simulink subsystem "Spline_Path_Following_sub"  (R2023b)
settings: Solver=VariableStepAuto  StartTime=0.0  StopTime=10.0  RelTol=1e-3
undefined symbols (not defined in the file): Spline_Lookahead_Dist
libraries: simulink x1
settings Model: Creator=ander  LastModifiedBy=ander

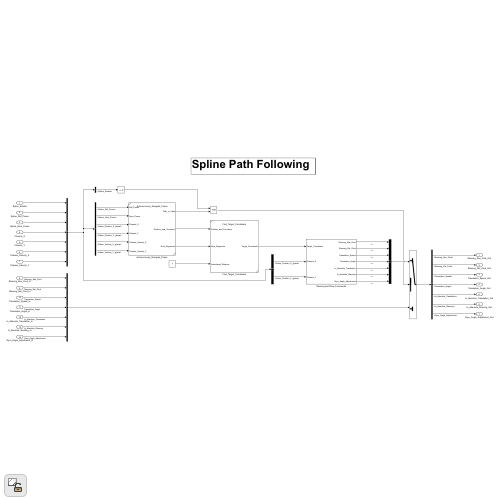
[thumbnail: Simulink's stored preview of the top-level diagram]
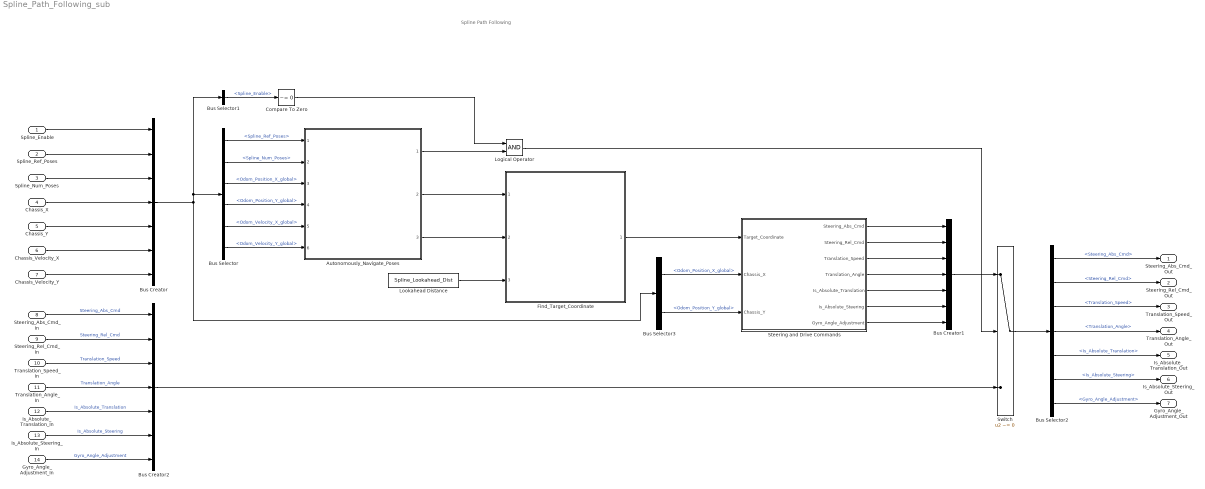
== system Spline_Path_Following_sub ==
  note: Spline Path Following
  Spline_Enable : Inport
  Spline_Ref_Poses : Inport  Port=2
  Spline_Num_Poses : Inport  Port=3
  Chassis_X : Inport  Port=4
  Chassis_Y : Inport  Port=5
  Chassis_Velocity_X : Inport  Port=6
  Chassis_Velocity_Y : Inport  Port=7
  Steering_Abs_Cmd_In : Inport  Port=8
  Steering_Rel_Cmd_In : Inport  Port=9
  Translation_Speed_In : Inport  Port=10
  Translation_Angle_In : Inport  Port=11
  Is_Absolute_Translation_In : Inport  Port=12
  Is_Absolute_Steering_In : Inport  Port=13
  Gyro_Angle_Adjustment_In : Inport  Port=14
  Autonomously_Navigate_Poses : Subsystem  ReferencedSubsystem=Autonomously_Navigate_Poses
  Bus Creator : BusCreator  Inputs=7
  Bus Creator1 : BusCreator  Inputs=7
  Bus Creator2 : BusCreator  Inputs=7
  Bus Selector : BusSelector  OutputSignals=Spline_Ref_Poses,Spline_Num_Poses,Odom_Position_X_global,Odom_Position_Y_global,Odom_Velocity_X_global,Odom_Velocity_Y_global
  Bus Selector1 : BusSelector  OutputSignals=Spline_Enable
  Bus Selector2 : BusSelector  OutputSignals=Steering_Abs_Cmd,Steering_Rel_Cmd,Translation_Speed,Translation_Angle,Is_Absolute_Translation,Is_Absolute_Steering,Gyro_Angle_Adjustment
  Bus Selector3 : BusSelector  OutputSignals=Odom_Position_X_global,Odom_Position_Y_global
  Compare To Zero : simulink/Logic and Bit Operations/Compare To Zero  relop=~=  OutDataTypeStr=boolean
  Find_Target_Coordinate : Subsystem  ReferencedSubsystem=Find_Target_Coordinate
  Logical Operator : Logic  AllPortsSameDT=off  OutDataTypeStr=boolean
  Lookahead Distance : Constant  Value=Spline_Lookahead_Dist
  Steering and Drive Commands : Subsystem
  Switch : Switch  Criteria=u2 ~= 0  SaturateOnIntegerOverflow=off  InputSameDT=off
  Steering_Abs_Cmd_Out : Outport
  Steering_Rel_Cmd_Out : Outport  Port=2
  Translation_Speed_Out : Outport  Port=3
  Translation_Angle_Out : Outport  Port=4
  Is_Absolute_Translation_Out : Outport  Port=5
  Is_Absolute_Steering_Out : Outport  Port=6
  Gyro_Angle_Adjustment_Out : Outport  Port=7
  wires:
  Chassis_Velocity_X/1 -> Bus Creator/6
  Spline_Enable/1 -> Bus Creator/1
  Spline_Ref_Poses/1 -> Bus Creator/2
  Spline_Num_Poses/1 -> Bus Creator/3
  Chassis_X/1 -> Bus Creator/4
  Chassis_Y/1 -> Bus Creator/5
  Gyro_Angle_Adjustment_In/1 -> Bus Creator2/7  "Gyro_Angle_Adjustment"
  Is_Absolute_Translation_In/1 -> Bus Creator2/5  "Is_Absolute_Translation"
  Translation_Speed_In/1 -> Bus Creator2/3  "Translation_Speed"
  Steering_Abs_Cmd_In/1 -> Bus Creator2/1  "Steering_Abs_Cmd"
  Chassis_Velocity_Y/1 -> Bus Creator/7
  Is_Absolute_Steering_In/1 -> Bus Creator2/6  "Is_Absolute_Steering"
  Translation_Angle_In/1 -> Bus Creator2/4  "Translation_Angle"
  Steering_Rel_Cmd_In/1 -> Bus Creator2/2  "Steering_Rel_Cmd"
  Autonomously_Navigate_Poses/2 -> Find_Target_Coordinate/1
  Autonomously_Navigate_Poses/1 -> Logical Operator/2
  Autonomously_Navigate_Poses/3 -> Find_Target_Coordinate/2
  Lookahead Distance/1 -> Find_Target_Coordinate/3
  Bus Creator/1 -> Bus Selector/1, Bus Selector1/1, Bus Selector3/1
  Bus Selector/2 -> Autonomously_Navigate_Poses/2  "<Spline_Num_Poses>"
  Bus Selector/3 -> Autonomously_Navigate_Poses/3  "<Odom_Position_X_global>"
  Bus Selector/1 -> Autonomously_Navigate_Poses/1  "<Spline_Ref_Poses>"
  Bus Selector/4 -> Autonomously_Navigate_Poses/4  "<Odom_Position_Y_global>"
  Bus Selector/5 -> Autonomously_Navigate_Poses/5  "<Odom_Velocity_X_global>"
  Bus Selector/6 -> Autonomously_Navigate_Poses/6  "<Odom_Velocity_Y_global>"
  Bus Selector1/1 -> Compare To Zero/1  "<Spline_Enable>"
  Switch/1 -> Bus Selector2/1
  Logical Operator/1 -> Switch/2
  Bus Selector2/1 -> Steering_Abs_Cmd_Out/1  "<Steering_Abs_Cmd>"
  Bus Selector2/2 -> Steering_Rel_Cmd_Out/1  "<Steering_Rel_Cmd>"
  Bus Selector2/3 -> Translation_Speed_Out/1  "<Translation_Speed>"
  Bus Selector2/4 -> Translation_Angle_Out/1  "<Translation_Angle>"
  Bus Selector2/5 -> Is_Absolute_Translation_Out/1  "<Is_Absolute_Translation>"
  Bus Selector2/6 -> Is_Absolute_Steering_Out/1  "<Is_Absolute_Steering>"
  Bus Selector2/7 -> Gyro_Angle_Adjustment_Out/1  "<Gyro_Angle_Adjustment>"
  Find_Target_Coordinate/1 -> Steering and Drive Commands/1(Target_Coordinate)
  Bus Creator2/1 -> Switch/3
  Steering and Drive Commands/5(Is_Absolute_Translation) -> Bus Creator1/5
  Steering and Drive Commands/4(Translation_Angle) -> Bus Creator1/4
  Steering and Drive Commands/6(Is_Absolute_Steering) -> Bus Creator1/6
  Steering and Drive Commands/3(Translation_Speed) -> Bus Creator1/3
  Steering and Drive Commands/7(Gyro_Angle_Adjustment) -> Bus Creator1/7
  Steering and Drive Commands/2(Steering_Rel_Cmd) -> Bus Creator1/2
  Steering and Drive Commands/1(Steering_Abs_Cmd) -> Bus Creator1/1
  Bus Creator1/1 -> Switch/1
  Bus Selector3/1 -> Steering and Drive Commands/2(Chassis_X)  "<Odom_Position_X_global>"
  Bus Selector3/2 -> Steering and Drive Commands/3(Chassis_Y)  "<Odom_Position_Y_global>"
  Compare To Zero/1 -> Logical Operator/1

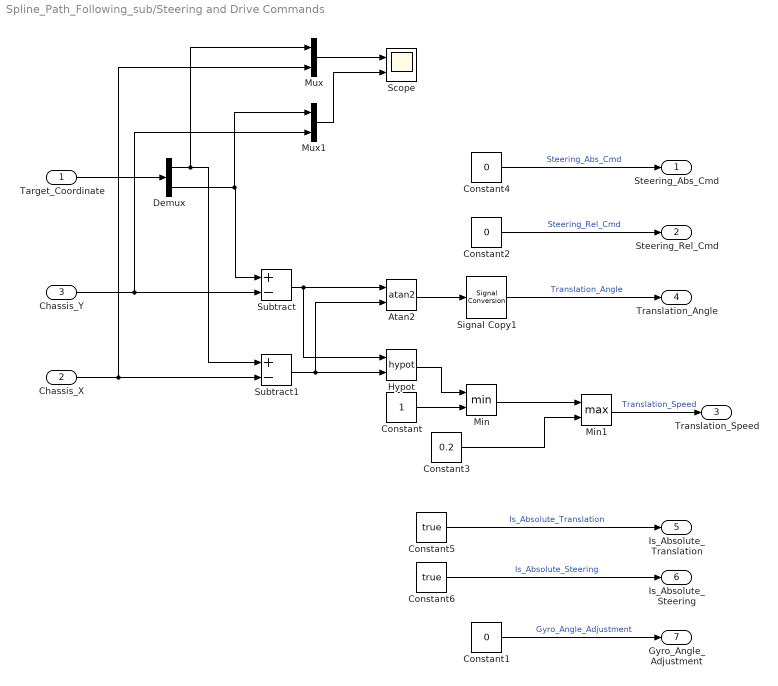
== system Spline_Path_Following_sub/Steering and Drive Commands ==
  Target_Coordinate : Inport
  Chassis_X : Inport  Port=2  OutDataTypeStr=double  Unit=m  PortDimensions=1
  Chassis_Y : Inport  Port=3  OutDataTypeStr=double  Unit=m  PortDimensions=1
  Atan2 : Trigonometry  Operator=atan2
  Constant : Constant
  Constant1 : Constant  Value=0
  Constant2 : Constant  Value=0
  Constant3 : Constant  Value=0.2
  Constant4 : Constant  Value=0
  Constant5 : Constant  Value=true
  Constant6 : Constant  Value=true
  Demux : Demux  Outputs=2
  Hypot : Math  Operator=hypot
  Min : MinMax  Inputs=2
  Min1 : MinMax  Function=max  Inputs=2
  Mux : Mux  Inputs=2
  Mux1 : Mux  Inputs=2
  Scope : Scope  NumInputPorts=2
  Signal Copy1 : SignalConversion  OverrideOpt=off
  Subtract : Sum  Inputs=+-
  Subtract1 : Sum  Inputs=+-
  Steering_Abs_Cmd : Outport
  Steering_Rel_Cmd : Outport  Port=2
  Translation_Speed : Outport  Port=3
  Translation_Angle : Outport  Port=4
  Is_Absolute_Translation : Outport  Port=5
  Is_Absolute_Steering : Outport  Port=6
  Gyro_Angle_Adjustment : Outport  Port=7
  wires:
  Constant3/1 -> Min1/2
  Min/1 -> Min1/1
  Mux1/1 -> Scope/2
  Mux/1 -> Scope/1
  Demux/1 -> Subtract1/1, Mux/1
  Target_Coordinate/1 -> Demux/1
  Subtract/1 -> Hypot/1, Atan2/1
  Subtract1/1 -> Hypot/2, Atan2/2
  Constant2/1 -> Steering_Rel_Cmd/1  "Steering_Rel_Cmd"
  Min1/1 -> Translation_Speed/1  "Translation_Speed"
  Constant6/1 -> Is_Absolute_Steering/1  "Is_Absolute_Steering"
  Constant5/1 -> Is_Absolute_Translation/1  "Is_Absolute_Translation"
  Chassis_X/1 -> Subtract1/2, Mux/2
  Constant4/1 -> Steering_Abs_Cmd/1  "Steering_Abs_Cmd"
  Hypot/1 -> Min/1
  Constant1/1 -> Gyro_Angle_Adjustment/1  "Gyro_Angle_Adjustment"
  Constant/1 -> Min/2
  Signal Copy1/1 -> Translation_Angle/1  "Translation_Angle"
  Demux/2 -> Subtract/1, Mux1/1
  Chassis_Y/1 -> Subtract/2, Mux1/2
  Atan2/1 -> Signal Copy1/1
